simulink model "odev21_simulasyon"  (R2019b)
settings: Solver=VariableStepAuto  StartTime=0.0  StopTime=100  RelTol=1e-3
settings Model: Creator=Mustafa Sezer  LastModifiedBy=Mustafa Sezer

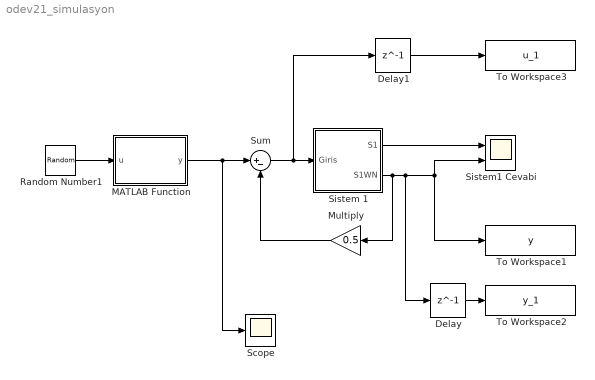
== system odev21_simulasyon ==
  Delay : Delay  DelayLength=1
  Delay1 : Delay  DelayLength=1
  MATLAB Function : MATLAB Function  TreatAsAtomicUnit=on
  Multiply : Gain  Gain=0.5
  Random Number1 : RandomNumber  Variance=0.5  Seed=1  SampleTime=0.1
  Scope : Scope
  Sistem 1 : Subsystem
  Sistem1 Cevabi : Scope  NumInputPorts=2
  Sum : Sum  Inputs=|+-
  To Workspace1 : ToWorkspace  VariableName=y  SaveFormat=Timeseries  SampleTime=-1
  To Workspace2 : ToWorkspace  VariableName=y_1  SaveFormat=Timeseries  SampleTime=-1
  To Workspace3 : ToWorkspace  VariableName=u_1  SaveFormat=Timeseries  SampleTime=-1
  wires:
  Sistem 1/1(S1) -> Sistem1 Cevabi/1
  Sistem 1/2(S1WN) -> Multiply/1, Delay/1, To Workspace1/1, Sistem1 Cevabi/2
  Delay/1 -> To Workspace2/1
  Sum/1 -> Delay1/1, Sistem 1/1(Giris)
  Multiply/1 -> Sum/2
  Delay1/1 -> To Workspace3/1
  MATLAB Function/1(y) -> Scope/1, Sum/1
  Random Number1/1 -> MATLAB Function/1(u)

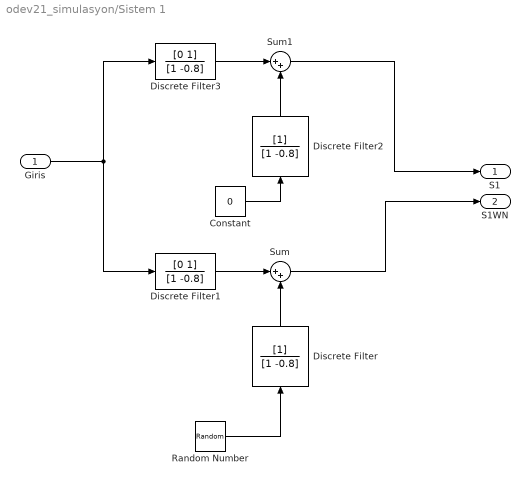
== system odev21_simulasyon/Sistem 1 ==
  Giris : Inport
  Constant : Constant  Value=0
  Discrete Filter : DiscreteFilter  Denominator=[1 -0.8]
  Discrete Filter1 : DiscreteFilter  Numerator=[0 1]  Denominator=[1 -0.8]
  Discrete Filter2 : DiscreteFilter  Denominator=[1 -0.8]
  Discrete Filter3 : DiscreteFilter  Numerator=[0 1]  Denominator=[1 -0.8]
  Random Number : RandomNumber  Seed=1  SampleTime=0.1
  Sum : Sum  Inputs=|++
  Sum1 : Sum  Inputs=|++
  S1 : Outport
  S1WN : Outport  Port=2
  wires:
  Discrete Filter/1 -> Sum/2
  Random Number/1 -> Discrete Filter/1
  Discrete Filter3/1 -> Sum1/1
  Constant/1 -> Discrete Filter2/1
  Discrete Filter1/1 -> Sum/1
  Sum/1 -> S1WN/1
  Discrete Filter2/1 -> Sum1/2
  Sum1/1 -> S1/1
  Giris/1 -> Discrete Filter1/1, Discrete Filter3/1

== matlab function odev21_simulasyon/MATLAB Function ==
  data: u input; y output
function y = fcn(u)
if u <= 0
    y = -0.5;
else
    y = 0.5;
end
end
